simulink model "AcceleratorFIR"  (R2019a)
settings: Solver=FixedStepAuto  StartTime=0.0  StopTime=20  FixedStep=step  RelTol=1e-3
model workspace (MAT data in the model file):
  step = 0.001
settings Model: OrderedModelArguments=off  Creator=EiLit  LastModifiedBy=EiLit
settings DataIOCC: ReturnWorkspaceOutputs=off
settings DebuggingCC: ReadBeforeWriteMsg=EnableAllAsWarning  WriteAfterWriteMsg=EnableAllAsWarning  WriteAfterReadMsg=EnableAllAsWarning  ArithmeticOperatorsInVariantConditions=warning

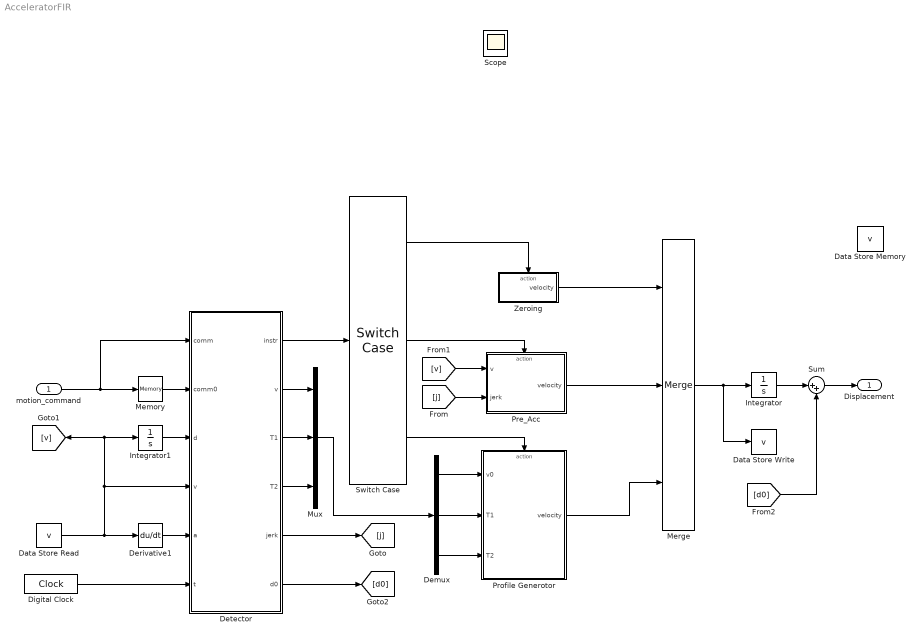
== system AcceleratorFIR ==
  motion_command : Inport
  Data Store Memory : DataStoreMemory  DataStoreName=v  ReadBeforeWriteMsg=warning  WriteAfterWriteMsg=warning  WriteAfterReadMsg=warning  ShowAdditionalParam=off  OutDataTypeStr=double
  Data Store Read : DataStoreRead  DataStoreName=v
  Data Store Write : DataStoreWrite  DataStoreName=v
  Demux : Demux  Outputs=3
  Derivative1 : Derivative
  Detector : MATLAB Function  TreatAsAtomicUnit=on
  Digital Clock : DigitalClock  SampleTime=step
  Integrator : Integrator
  Integrator1 : Integrator
  Memory : Memory  InitialCondition=[0 0 0 0]
  Merge : Merge  Inputs=3  InitialOutput=0
  Mux : Mux  Inputs=3
  Pre_Acc : Subsystem  TreatAsAtomicUnit=on
  Profile Generotor : Subsystem
  Sum : Sum  Inputs=|++
  Switch Case : SwitchCase  CaseConditions={0,1,2}  ShowDefaultCase=off
  Zeroing : Subsystem  TreatAsAtomicUnit=on
  Displacement : Outport
  Scope : Scope
  wires:
  motion_command/1 -> Detector/1(comm), Memory/1
  Memory/1 -> Detector/2(comm0)
  Digital Clock/1 -> Detector/6(t)
  Detector/1(instr) -> Switch Case/1
  Switch Case/1 -> Zeroing/Action
  Detector/2(v) -> Mux/1
  Detector/3(T1) -> Mux/2
  Detector/4(T2) -> Mux/3
  Demux/1 -> Profile Generotor/1(v0)
  Demux/2 -> Profile Generotor/2(T1)
  Demux/3 -> Profile Generotor/3(T2)
  Mux/1 -> Demux/1
  Switch Case/3 -> Profile Generotor/Action
  Switch Case/2 -> Pre_Acc/Action
  Merge/1 -> Integrator/1, Data Store Write/1
  Zeroing/1(velocity) -> Merge/1
  Pre_Acc/1(velocity) -> Merge/2
  Profile Generotor/1(velocity) -> Merge/3
  Detector/5(jerk) -> [j]
  Data Store Read/1 -> Derivative1/1, Detector/4("v "), [v], Integrator1/1
  Derivative1/1 -> Detector/5(a)
  [j] -> Pre_Acc/2(jerk)
  [v] -> Pre_Acc/1(v)
  Integrator/1 -> Sum/1
  Sum/1 -> Displacement/1
  Detector/6(d0) -> [d0]
  [d0] -> Sum/2
  Integrator1/1 -> Detector/3(d)

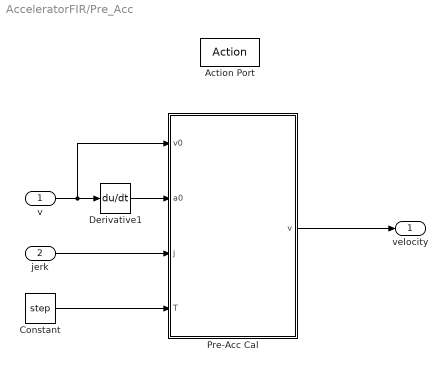
== system AcceleratorFIR/Pre_Acc ==
  v : Inport
  jerk : Inport  Port=2
  Action Port : ActionPort  ActionPortLabel=case [ 1 ]:
  Constant : Constant  Value=step
  Derivative1 : Derivative
  Pre-Acc Cal : MATLAB Function  TreatAsAtomicUnit=on
  velocity : Outport
  wires:
  Pre-Acc Cal/1(v) -> velocity/1
  v/1 -> Pre-Acc Cal/1(v0), Derivative1/1
  Derivative1/1 -> Pre-Acc Cal/2(a0)
  jerk/1 -> Pre-Acc Cal/3(j)
  Constant/1 -> Pre-Acc Cal/4(T)

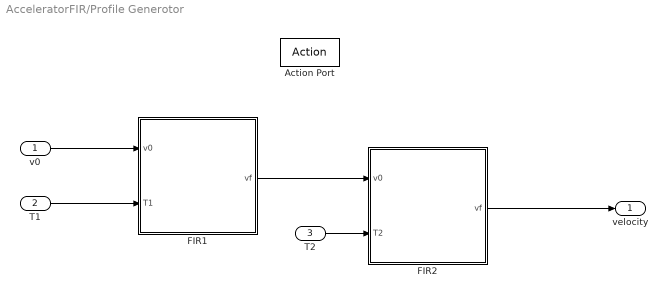
== system AcceleratorFIR/Profile Generotor ==
  v0 : Inport
  T1 : Inport  Port=2
  T2 : Inport  Port=3
  Action Port : ActionPort  ActionPortLabel=case [ 2 ]:
  FIR1 : Subsystem
  FIR2 : Subsystem
  velocity : Outport
  wires:
  FIR2/1(vf) -> velocity/1
  v0/1 -> FIR1/1(v0)
  T2/1 -> FIR2/2(T2)
  T1/1 -> FIR1/2(T1)
  FIR1/1(vf) -> FIR2/1(v0)

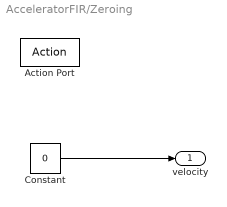
== system AcceleratorFIR/Zeroing ==
  Action Port : ActionPort  ActionPortLabel=case [ 0 ]:
  Constant : Constant  Value=0
  velocity : Outport
  wires:
  Constant/1 -> velocity/1

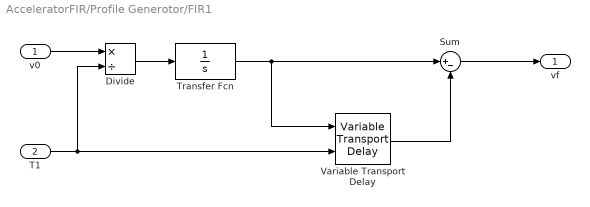
== system AcceleratorFIR/Profile Generotor/FIR1 ==
  v0 : Inport
  T1 : Inport  Port=2
  Divide : Product  Inputs=*/
  Sum : Sum  Inputs=|+-
  Transfer Fcn : TransferFcn  Denominator=[1 0]
  Variable Transport Delay : VariableTransportDelay  MaximumDelay=10
  vf : Outport
  wires:
  v0/1 -> Divide/1
  Divide/1 -> Transfer Fcn/1
  Transfer Fcn/1 -> Variable Transport Delay/1, Sum/1
  Variable Transport Delay/1 -> Sum/2
  Sum/1 -> vf/1
  T1/1 -> Variable Transport Delay/2, Divide/2

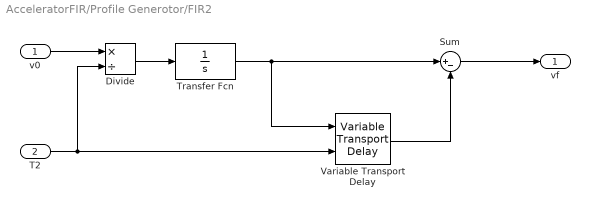
== system AcceleratorFIR/Profile Generotor/FIR2 ==
  v0 : Inport
  T2 : Inport  Port=2
  Divide : Product  Inputs=*/
  Sum : Sum  Inputs=|+-
  Transfer Fcn : TransferFcn  Denominator=[1 0]
  Variable Transport Delay : VariableTransportDelay  MaximumDelay=10
  vf : Outport
  wires:
  v0/1 -> Divide/1
  Divide/1 -> Transfer Fcn/1
  Transfer Fcn/1 -> Variable Transport Delay/1, Sum/1
  Variable Transport Delay/1 -> Sum/2
  Sum/1 -> vf/1
  T2/1 -> Variable Transport Delay/2, Divide/2

== matlab function AcceleratorFIR/Pre_Acc/Pre-Acc Cal ==
  data: v output; v0 input; a0 input; j input; T input
function v = fcn(v0,a0,j,T)
% This function used to calculate the pre-Acc displacement;
if a0*(a0+j*T) > 0                                      % If is deccelerated to 0.
    v = v0 + a0*T + 1/2*j*T^2;
else
    v = v0 + a0*T + 1/2*(0-a0)/T*T^2;
end

== matlab function AcceleratorFIR/Detector ==
  data: instr output; comm input; v output; T1 output; T2 output; comm0 input; d input; v input; a input; t input; jerk output; d0 output
function [instr, v, T1, T2, jerk, d0] = fcn(comm, comm0, d, v, a, t)
%% Initialization
persistent pre_flag preed_flag Acc_flag cal_flag t1A t2 t1D

if isempty(pre_flag)
    pre_flag = 0;
end
if isempty(preed_flag)
    preed_flag = 1;
end
if isempty(Acc_flag)
    Acc_flag = 1;
end
if isempty(cal_flag)
    cal_flag = 0;
end
if isempty(t1A)
    t1A = 0;
end
if isempty(t2)
    t2 = 0;
end
if isempty(t1D)
    t1D = 0;
end

%% comm changed
if ~(comm==comm0)
    if a ~= 0               % if nedd pre_flag
        pre_flag = 1;
        preed_flag = 0;
    end
end

%% the pre-acc phase
if pre_flag == 1
    if a ~= 0
        jerk = -a/abs(a) * abs(comm(4));
        instr = 1;
        d0 = 0;
    else
        pre_flag = 0;
        preed_flag = 1;
    end
end

%% acceleration phase
if pre_flag == 0
    if cal_flag == 0
        cal_flag = 1;
        t0 = t;                     % Reset the time
        t2 = comm(3)/comm(4);
        deltv = comm(3)^2/(2*comm(4));
        t1A = (comm(2)-deltv-v) / comm(3);
        t1D = 
    end
    if Acc_flag == 1
